simulink subsystem "Piero"  (R2023b)
settings: Solver=VariableStepAuto  StartTime=0.0  StopTime=10.0  RelTol=1e-3
settings Model: Creator=Usuario_UMA  LastModifiedBy=Manuel

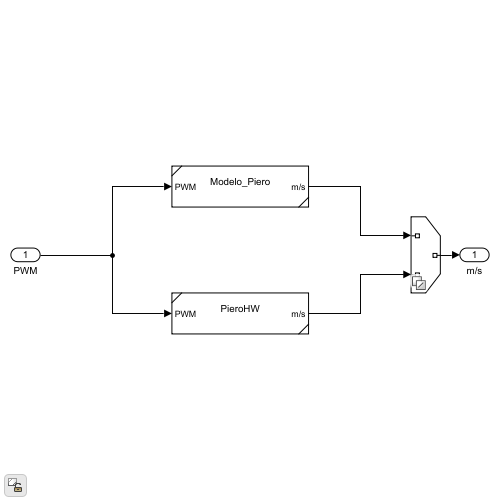
[thumbnail: Simulink's stored preview of the top-level diagram]
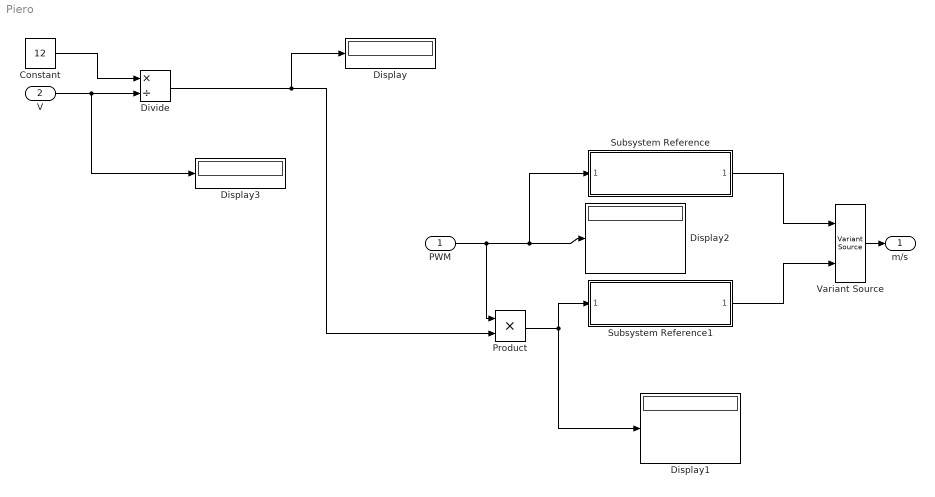
== system Piero ==
  PWM : Inport
  V : Inport  Port=2
  Constant : Constant  Value=12
  Display{,1..3} (4 alike) : Display
  Divide : Product  Inputs=*/
  Product : Product
  Subsystem Reference : Subsystem  ReferencedSubsystem=Modelo_Piero
  Subsystem Reference1 : Subsystem  ReferencedSubsystem=PieroHW
  Variant Source : VariantSource  VariantControlMode=sim codegen switching
  m/s : Outport
  wires:
  Subsystem Reference1/1 -> Variant Source/2
  Subsystem Reference/1 -> Variant Source/1
  Variant Source/1 -> m/s/1
  PWM/1 -> Product/1, Subsystem Reference/1, Display2/1
  V/1 -> Divide/2, Display3/1
  Constant/1 -> Divide/1
  Product/1 -> Display1/1, Subsystem Reference1/1
  Divide/1 -> Product/2, Display/1
